simulink model "BalancingRobotModel"  (R2020b)
settings: Solver=VariableStepAuto  StartTime=0.0  StopTime=10.0  RelTol=1e-3
values from neighbouring files (symbols this model uses):
  A = [0, 0 ,1, 0 ... (first row only)    [BalancingRobotSystem.m]    (also in ControlBootcampModel.m = [0 1 0 0)
  Ad = sys_d.a    [BalancingRobotSystem.m]
  B = [0; 0; 1/mc; 1/(L*mc)]    [BalancingRobotSystem.m]    (also in ControlBootcampModel.m = [0; 1/M; 0; s*1/(M*L)])
  Bd = sys_d.b    [BalancingRobotSystem.m]
  C = [1 0 0 0]    [BalancingRobotSystem.m]    (also in ControlBootcampModel.m = [1 1 1 1])
  Cd = sys_d.c    [BalancingRobotSystem.m]
  K_discLQR = dlqr(Ad,Bd,Q,R)    [BalancingRobotSystem.m]
  Ob = acker(Ad',Cd',disc_PolesOb)    [BalancingRobotSystem.m]
  Ts = 0.01    [BalancingRobotSystem.m]
  x0 = [0; 5*pi/180; 0; 0;]    [BalancingRobotSystem.m]    (also in ControlBootcampModel.m = [0; 0; pi; .5])
settings Model: Creator=Nikola  LastModifiedBy=Nikola

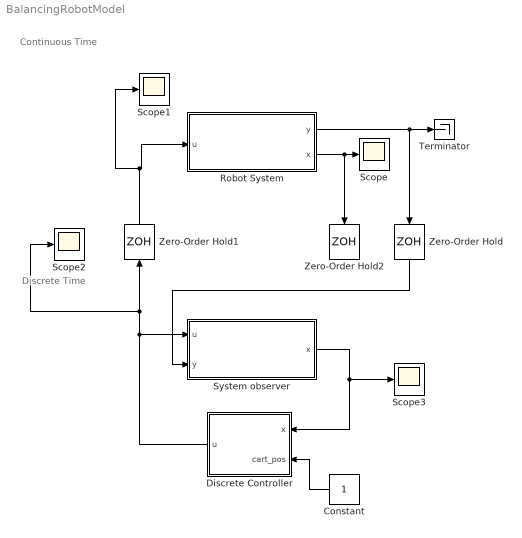
== system BalancingRobotModel ==
  note: Continuous Time
  note: Discrete Time
  Constant : Constant
  Discrete Controller : Subsystem
  Robot System : Subsystem
  Scope{,1..3} (4 alike) : Scope
  System observer : Subsystem
  Terminator : Terminator
  Zero-Order Hold : ZeroOrderHold  SampleTime=Ts
  Zero-Order Hold1 : ZeroOrderHold  SampleTime=Ts
  Zero-Order Hold2 : ZeroOrderHold  SampleTime=Ts
  wires:
  Robot System/1(y) -> Terminator/1, Zero-Order Hold/1
  Robot System/2(x) -> Zero-Order Hold2/1, Scope/1
  Discrete Controller/1(u) -> System observer/1(u), Scope2/1, Zero-Order Hold1/1
  Constant/1 -> Discrete Controller/2(cart_pos)
  Zero-Order Hold1/1 -> Robot System/1(u), Scope1/1
  Zero-Order Hold/1 -> System observer/2(y)
  System observer/1(x) -> Discrete Controller/1(x), Scope3/1

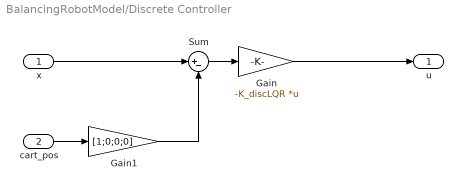
== system BalancingRobotModel/Discrete Controller ==
  x : Inport
  cart_pos : Inport  Port=2
  Gain : Gain  Gain=-K_discLQR  Multiplication=Matrix(K*u)
  Gain1 : Gain  Gain=[1;0;0;0]
  Sum : Sum  Inputs=|+-
  u : Outport
  wires:
  Gain/1 -> u/1
  x/1 -> Sum/1
  cart_pos/1 -> Gain1/1
  Sum/1 -> Gain/1
  Gain1/1 -> Sum/2

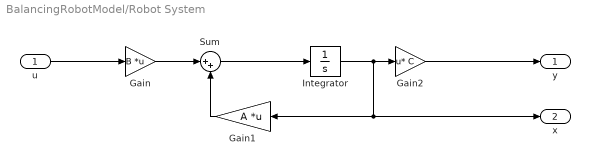
== system BalancingRobotModel/Robot System ==
  u : Inport
  Gain : Gain  Gain=B  Multiplication=Matrix(K*u)
  Gain1 : Gain  Gain=A  Multiplication=Matrix(K*u) (u vector)
  Gain2 : Gain  Gain=C  Multiplication=Matrix(u*K)
  Integrator : Integrator  InitialCondition=x0
  Sum : Sum  Inputs=|++
  y : Outport
  x : Outport  Port=2
  wires:
  Gain2/1 -> y/1
  Sum/1 -> Integrator/1
  Gain1/1 -> Sum/2
  Integrator/1 -> Gain2/1, x/1, Gain1/1
  u/1 -> Gain/1
  Gain/1 -> Sum/1

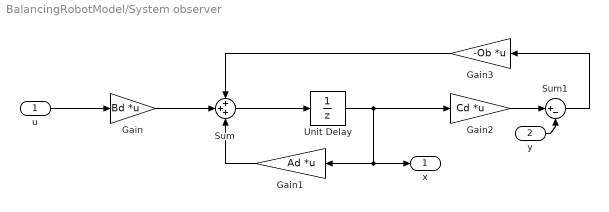
== system BalancingRobotModel/System observer ==
  u : Inport
  y : Inport  Port=2
  Gain : Gain  Gain=Bd  Multiplication=Matrix(K*u)
  Gain1 : Gain  Gain=Ad  Multiplication=Matrix(K*u) (u vector)
  Gain2 : Gain  Gain=Cd  Multiplication=Matrix(K*u)
  Gain3 : Gain  Gain=-Ob  Multiplication=Matrix(K*u)
  Sum : Sum  Inputs=+++
  Sum1 : Sum  Inputs=|+-
  Unit Delay : UnitDelay  InitialCondition=x0*0  SampleTime=-1  HasFrameUpgradeWarning=on
  x : Outport
  wires:
  Gain2/1 -> Sum1/1
  Sum/1 -> Unit Delay/1
  Unit Delay/1 -> Gain2/1, x/1, Gain1/1
  u/1 -> Gain/1
  y/1 -> Sum1/2
  Sum1/1 -> Gain3/1
  Gain1/1 -> Sum/3
  Gain/1 -> Sum/2
  Gain3/1 -> Sum/1
